simulink model "bms"  (R2025b)
settings: Solver=VariableStepAuto  StartTime=0.0  StopTime=3600  RelTol=1e-3
libraries: simulink x2, SignalEditorBlockLib x1

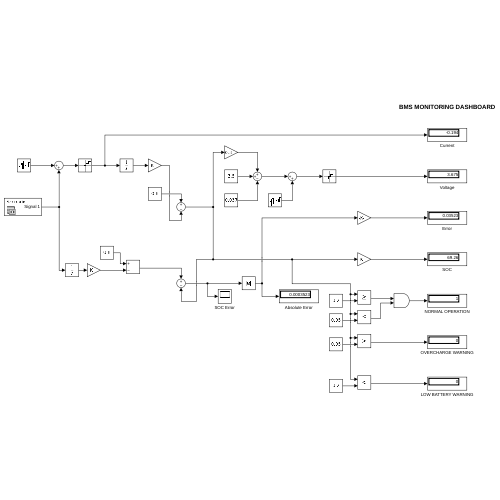
[thumbnail: Simulink's stored preview of the top-level diagram]
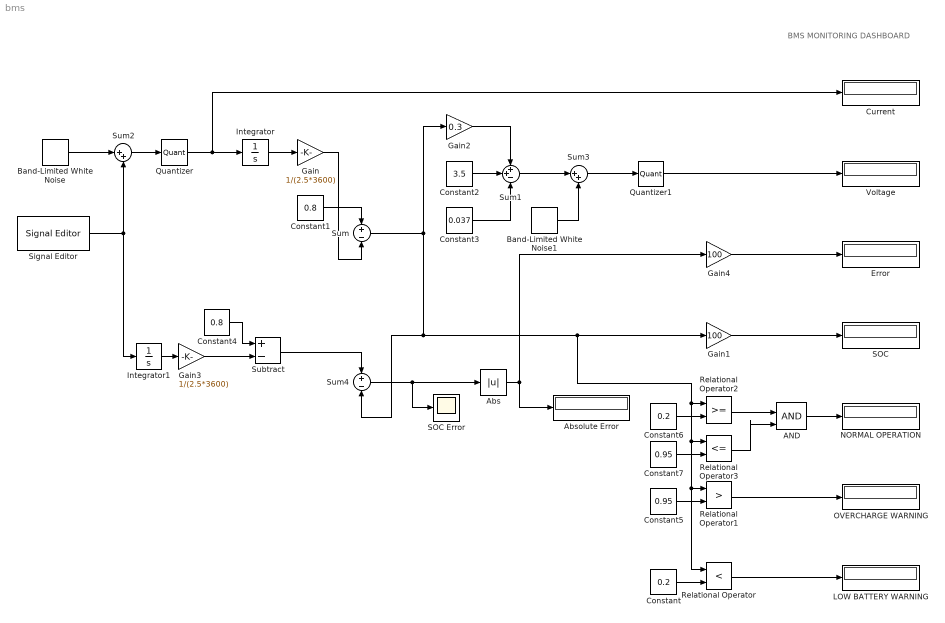
== system bms ==
  note: BMS MONITORING DASHBOARD
  AND : Logic  IconShape=distinctive  AllPortsSameDT=off  OutDataTypeStr=boolean
  Abs : Abs  SaturateOnIntegerOverflow=off
  Absolute Error : Display
  Band-Limited White Noise : simulink/Sources/Band-Limited White Noise  Cov=0.001  Ts=1  seed=[23341]
  Band-Limited White Noise1 : simulink/Sources/Band-Limited White Noise  Cov=0.0001  Ts=1  seed=[23342]
  Constant : Constant  Value=0.2
  Constant1 : Constant  Value=0.8
  Constant2 : Constant  Value=3.5
  Constant3 : Constant  Value=0.037
  Constant4 : Constant  Value=0.8
  Constant5 : Constant  Value=0.95
  Constant6 : Constant  Value=0.2
  Constant7 : Constant  Value=0.95
  Current : Display
  Error : Display
  Gain : Gain  Gain=1/(2.5*3600)
  Gain1 : Gain  Gain=100
  Gain2 : Gain  Gain=0.3
  Gain3 : Gain  Gain=1/(2.5*3600)
  Gain4 : Gain  Gain=100
  Integrator : Integrator
  Integrator1 : Integrator
  LOW BATTERY WARNING : Display
  NORMAL OPERATION : Display
  OVERCHARGE WARNING : Display
  Quantizer : Quantizer  QuantizationInterval=0.001
  Quantizer1 : Quantizer  QuantizationInterval=0.001
  Relational Operator : RelationalOperator  Operator=<  OutDataTypeStr=boolean  RndMeth=Simplest  InputSameDT=off
  Relational Operator1 : RelationalOperator  Operator=>  OutDataTypeStr=boolean  RndMeth=Simplest  InputSameDT=off
  Relational Operator2 : RelationalOperator  OutDataTypeStr=boolean  RndMeth=Simplest  InputSameDT=off
  Relational Operator3 : RelationalOperator  Operator=<=  OutDataTypeStr=boolean  RndMeth=Simplest  InputSameDT=off
  SOC : Display
  SOC Error : Scope
      settings: ActiveDisplayYMinimum=-1.6317917916666667  ActiveDisplayYMaximum=-1.3138738750000016  DataLoggingVariableName=ScopeData3
  Signal Editor : SignalEditorBlockLib/Signal Editor  FileName=Dynamic_Load_Profile.mat  ActiveScenario=Scenario  ActiveSignal=Signal 1  IsBus=off  OutputBusObjectStr=Bus: BusObject  SampleTime=1  ZeroCross=off  OutputAfterFinalValue=Setting to zero  Unit=inherit  PreserveSignalName=on  ApplySigPropsToAllScenarios=on  ApplySigPropsToAllSignals=off  SignalPropertySource=Dialog parameters
  Subtract : Sum  Inputs=+-
  Sum : Sum  Inputs=+-
  Sum1 : Sum  Inputs=++-
  Sum2 : Sum  Inputs=|++
  Sum3 : Sum  Inputs=|++
  Sum4 : Sum  Inputs=+-
  Voltage : Display
  wires:
  Integrator/1 -> Gain/1
  Gain/1 -> Sum/2
  Constant1/1 -> Sum/1
  Sum/1 -> Gain2/1, Sum4/2, Relational Operator/1, Relational Operator1/1, Relational Operator3/1, Relational Operator2/1, Gain1/1
  Gain2/1 -> Sum1/1
  Constant2/1 -> Sum1/2
  Constant3/1 -> Sum1/3
  Signal Editor/1 -> Integrator1/1, Sum2/2
  Band-Limited White Noise/1 -> Sum2/1
  Sum2/1 -> Quantizer/1
  Quantizer/1 -> Current/1, Integrator/1
  Band-Limited White Noise1/1 -> Sum3/2
  Sum1/1 -> Sum3/1
  Sum3/1 -> Quantizer1/1
  Quantizer1/1 -> Voltage/1
  Integrator1/1 -> Gain3/1
  Gain3/1 -> Subtract/2
  Subtract/1 -> Sum4/1
  Abs/1 -> Gain4/1, Absolute Error/1
  Constant4/1 -> Subtract/1
  Sum4/1 -> SOC Error/1, Abs/1
  Constant/1 -> Relational Operator/2
  Relational Operator/1 -> LOW BATTERY WARNING/1
  Constant5/1 -> Relational Operator1/2
  Relational Operator1/1 -> OVERCHARGE WARNING/1
  Constant6/1 -> Relational Operator2/2
  Constant7/1 -> Relational Operator3/2
  Relational Operator2/1 -> AND/1
  Relational Operator3/1 -> AND/2
  AND/1 -> NORMAL OPERATION/1
  Gain1/1 -> SOC/1
  Gain4/1 -> Error/1
